simulink model "Luenberger_NonLinear_Final"  (R2019b)
settings: Solver=VariableStepAuto  StartTime=0.0  StopTime=200  RelTol=1e-3
undefined symbols (not defined in the file): A, B, C
libraries: eeLuenbergerObserver x1
settings Model: Creator=Pranali  LastModifiedBy=shubh
settings DataIOCC: ReturnWorkspaceOutputs=off
settings DebuggingCC: ArithmeticOperatorsInVariantConditions=warning
settings SFSimCC: CustomCodeUndefinedFunction=UseInterfaceOnly

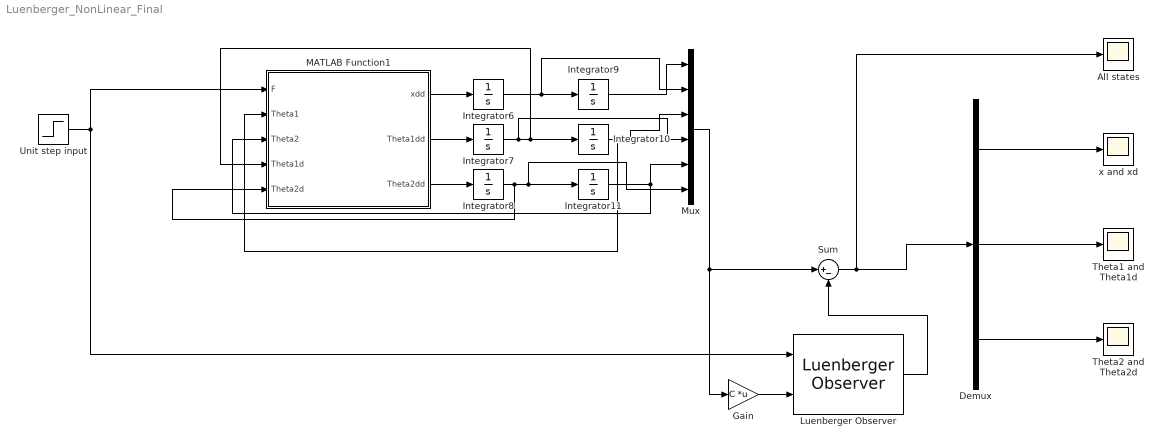
== system Luenberger_NonLinear_Final ==
  All states : Scope
  Demux : Demux  Outputs=3
  Gain : Gain  Gain=C  Multiplication=Matrix(K*u)
  Integrator{6..11} (6 alike) : Integrator
  "Luenberger Observer " : eeLuenbergerObserver/Luenberger Observer  StateSpaceType=Continuous-time  Ad=A  Bd=B  Cd=C  Dd=D  A=A  B=B  C=C  D=[0]  ObserverDesign=Observer gain  Ld=L  DesiredEigenvalues=[-0.2 -0.3 -0.4 -0.5 -0.6 -0.7]  x0="[0.5 0  pi/6 0  pi/6 0]"  Tsd=0.1  Ts=0.1
      settings: SourceProductName=Simscape Electrical  SourceProductBaseCode=PS
  MATLAB Function1 : MATLAB Function  TreatAsAtomicUnit=on
  Mux : Mux  Inputs=6
  Sum : Sum  Inputs=|+-
  Theta1 and Theta1d : Scope
  Theta2 and Theta2d : Scope
  "Unit step input " : Step  Time=10  SampleTime=0
  x and xd : Scope
  wires:
  MATLAB Function1/2(Theta1dd) -> Integrator7/1
  Integrator7/1 -> Mux/4, MATLAB Function1/4(Theta1d), Integrator10/1
  MATLAB Function1/1(xdd) -> Integrator6/1
  Integrator9/1 -> Mux/1
  MATLAB Function1/3(Theta2dd) -> Integrator8/1
  Integrator8/1 -> MATLAB Function1/5(Theta2d), Mux/6, Integrator11/1
  Integrator6/1 -> Mux/2, Integrator9/1
  Mux/1 -> Gain/1, Sum/1
  Sum/1 -> Demux/1, All states/1
  Demux/1 -> x and xd/1
  Demux/3 -> Theta2 and Theta2d/1
  Gain/1 -> "Luenberger Observer "/2
  "Luenberger Observer "/1 -> Sum/2
  "Unit step input "/1 -> MATLAB Function1/1(F), "Luenberger Observer "/1
  Integrator10/1 -> Mux/3, MATLAB Function1/2(Theta1)
  Integrator11/1 -> MATLAB Function1/3(Theta2), Mux/5
  Demux/2 -> Theta1 and Theta1d/1

== matlab function Luenberger_NonLinear_Final/MATLAB Function1 ==
  data: F input; Theta1 input; Theta2 input; xdd output; Theta1d input; Theta2d input; Theta1dd output; Theta2dd output
function [xdd,Theta1dd,Theta2dd] = NL_Luenberger(F,Theta1,Theta2,Theta1d,Theta2d)

l1 = 20; 
l2 = 10; 
m1 = 100; 
m2 = 100; 
M = 1000; 
g = 9.81;
%% x_ddot equation 
xdd = (F - m1*cos(Theta1)*sin(Theta1)*g - m2*cos(Theta2)*sin(Theta2)*g - m1*l1*(Theta1d^2)*(sin(Theta1)) - m2*l2*(Theta2d^2)*(sin(Theta2)))/(M + m1*(sin(Theta1)^2) + m2*(sin(Theta2)^2));

%% Theta1_ddot equation
Theta1dd = (xdd*cos(Theta1) - g*sin(Theta1))/l1;

%% Theta2_ddot equation
Theta2dd = (xdd*cos(Theta2) - g*sin(Theta2))/l2;

end
